simulink model "dog_fsm"  (R2023a)
settings: Solver=FixedStepDiscrete  StartTime=0.0  StopTime=10.0  FixedStep=0.1  RelTol=1e-3  EnableMultiTasking=on
settings Model: Creator=yaboi  LastModifiedBy=yaboi
settings SolverCC: AlgebraicLoopSolver=TrustRegion  AutoInsertRateTranBlk=on
settings DataIOCC: LimitDataPoints=on
settings OptimizationCC: LifeSpan=inf
settings DebuggingCC: UnconnectedInputMsg=warning  UnconnectedOutputMsg=warning  UnconnectedLineMsg=warning  AllowSymbolicDim=off  SFUnexpectedBacktrackingDiag=warning  SFNoUnconditionalDefaultTransitionDiag=warning  SFExecutionAtInitializationDiag=none  ArithmeticOperatorsInVariantConditions=warning
settings ModelReferenceCC: EnableRefExpFcnMdlSchedulingChecks=on
settings SFSimCC: SimUseLocalCustomCode=off  CustomCodeUndefinedFunction=UseInterfaceOnly
settings RTWCC: RTWUseLocalCustomCode=off  DLArmComputeVersion=19.05
settings CodeAppCC: StateflowObjectComments=on
settings GRTTargetCC: TargetLangStandard=C89/C90 (ANSI)
settings ConfigComp: CovMetricSettings=dw  CovSaveCumulativeToWorkspaceVar=on  CovSaveSingleToWorkspaceVar=on  CovExternalEMLEnable=off  CovSFcnEnable=off

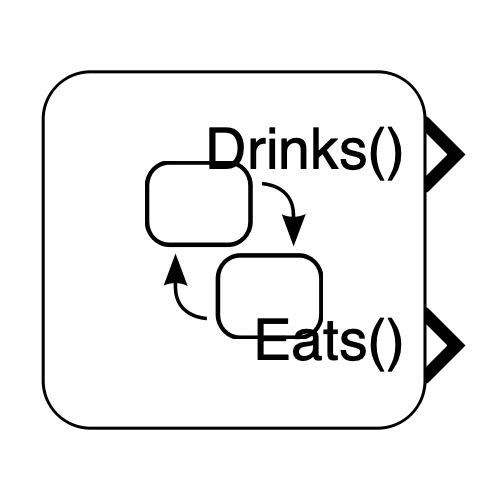
[thumbnail: Simulink's stored preview of the top-level diagram]
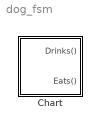
== system dog_fsm ==
  Chart : Stateflow chart  TreatAsAtomicUnit=on

== stateflow chart dog_fsm/Chart ==
  state Thirsty
  state Full
    i = i + 1
  state Hungry
  Full -> Thirsty [order 2] : [i > 5]
  Thirsty -> Full : Drinks
      | [1]
      | {i = 0}
  (default) -> Full
  Full -> Hungry [order 1] : [i > 5]
  Hungry -> Full : Eats
      | [1]
      | {i = 0}
  data: i local =0
  events: Drinks output FUNCTION_CALL_EVENT; Eats output FUNCTION_CALL_EVENT
